simulink model "cartpole"  (R2019b)
settings: Solver=ode15s  StartTime=0.0  StopTime=10  MaxStep=0.01  RelTol=1e-3  EnableMultiTasking=on
values from neighbouring files (symbols this model uses):
  cartpole_init_pose = [-(ground.w/2-1) tire.r+ground.l/2 0]    [cartpole_conf.m]
  g = 9.81    [cartpole_conf.m]
  m_cart = body.m + 2*tire.m + 4*omni.m    [cartpole_conf.m]
  max_steer = 0.42    [cartpole_conf.m]
  max_v = 1    [cartpole_conf.m]
  path = [4.0 0.0 2.0]    [cartpole_conf.m]
  tread = tire.l + body.h    [cartpole_conf.m]
  waypoint_length = 0.05    [cartpole_conf.m]
undefined symbols (not defined in the file or in its folder): body, Body, ground, Ground, LBomni, LCtire, LFomni, omni, RBomni, RCtire, RFomni, sigbuilder_block, stick, Stick, tire, Wall1, Wall2, Wall3, Wall4, X, Y, Z
libraries: sm_lib x106, nesl_utility x18, simulink x5
(part 4 of 4)

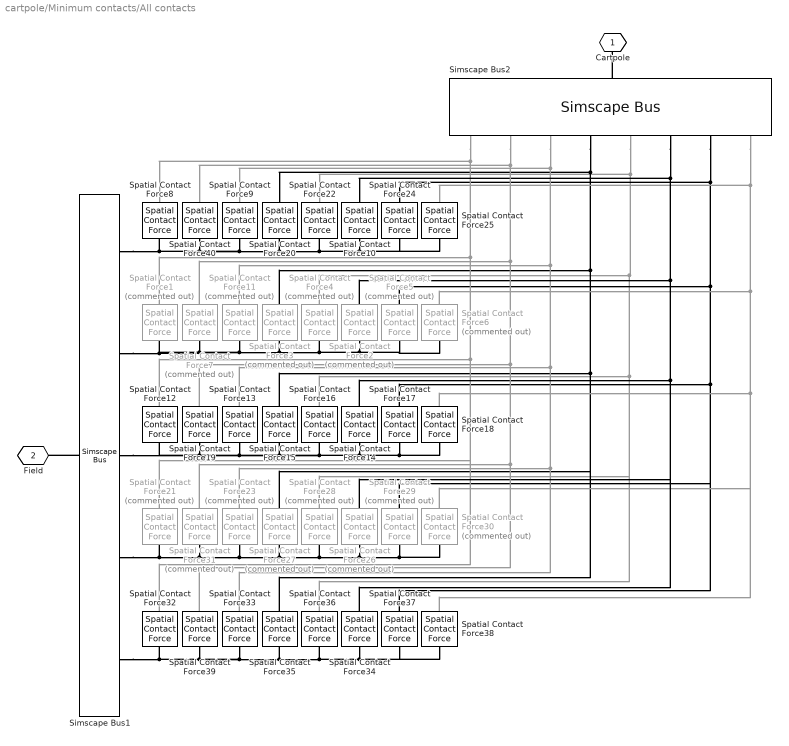
== system cartpole/Minimum contacts/All contacts ==
  Simscape Bus1 : SimscapeBus  HierarchyStrings=Wall1;Wall2;Wall3;Wall4;Ground
  Simscape Bus2 : SimscapeBus  HierarchyStrings=Stick;LFomni;LCtire;LBomni;RFomni;RCtire;RBomni;Body
  Spatial Contact Force{1..7,11,21,23,26..31} (16 alike) : sm_lib/Forces and Torques/Spatial Contact Force  Commented=on  CoefficientOfDynamicFriction=0.5  CoefficientOfStaticFriction=0.7  NormalDamping=1e3  NormalDampingUnits=N/(m/s)  NormalStiffness=1e6  NormalStiffnessUnits=N/m  FrictionalCriticalVelocity=1e-3  FrictionalCriticalVelocityUnits=m/s  SenseFrictionalForceMagnitude=off  SenseNormalForceMagnitude=off  SenseSeparationDistance=off  NormalTransitionRegionWidth=1e-4  NormalTransitionRegionWidthUnits=m  FrictionType=SmoothStickSlip
      settings: SourceProductName=Simscape Multibody
  Spatial Contact Force{8..10,12..20,22,24..25,32..40} (24 alike) : sm_lib/Forces and Torques/Spatial Contact Force  CoefficientOfDynamicFriction=0.5  CoefficientOfStaticFriction=0.7  NormalDamping=1e3  NormalDampingUnits=N/(m/s)  NormalStiffness=1e6  NormalStiffnessUnits=N/m  FrictionalCriticalVelocity=1e-3  FrictionalCriticalVelocityUnits=m/s  SenseFrictionalForceMagnitude=off  SenseNormalForceMagnitude=off  SenseSeparationDistance=off  NormalTransitionRegionWidth=1e-4  NormalTransitionRegionWidthUnits=m  FrictionType=SmoothStickSlip
      settings: SourceProductName=Simscape Multibody
  Cartpole : PMIOPort  Side=Right
  Field : PMIOPort  Port=2  Side=Left
  connections:
  Spatial Contact Force4/RConn1 -- Spatial Contact Force36/RConn1 -- Spatial Contact Force28/RConn1 -- Spatial Contact Force16/RConn1 -- Simscape Bus2/LConn5 -- Spatial Contact Force22/RConn1
  Spatial Contact Force1/LConn1 -- Simscape Bus1/LConn2 -- Spatial Contact Force7/LConn1 -- Spatial Contact Force11/LConn1 -- Spatial Contact Force3/LConn1 -- Spatial Contact Force2/LConn1 -- Spatial Contact Force6/LConn1 -- Spatial Contact Force5/LConn1 -- Spatial Contact Force4/LConn1
  Spatial Contact Force17/RConn1 -- Spatial Contact Force5/RConn1 -- Simscape Bus2/LConn7 -- Spatial Contact Force24/RConn1 -- Spatial Contact Force37/RConn1 -- Spatial Contact Force29/RConn1
  Spatial Contact Force15/RConn1 -- Spatial Contact Force3/RConn1 -- Simscape Bus2/LConn4 -- Spatial Contact Force20/RConn1 -- Spatial Contact Force35/RConn1 -- Spatial Contact Force27/RConn1
  Spatial Contact Force32/LConn1 -- Simscape Bus1/LConn5 -- Spatial Contact Force34/LConn1 -- Spatial Contact Force38/LConn1 -- Spatial Contact Force37/LConn1 -- Spatial Contact Force36/LConn1 -- Spatial Contact Force35/LConn1 -- Spatial Contact Force33/LConn1 -- Spatial Contact Force39/LConn1
  Spatial Contact Force6/RConn1 -- Spatial Contact Force38/RConn1 -- Spatial Contact Force30/RConn1 -- Spatial Contact Force18/RConn1 -- Simscape Bus2/LConn8 -- Spatial Contact Force25/RConn1
  Spatial Contact Force1/RConn1 -- Spatial Contact Force32/RConn1 -- Spatial Contact Force21/RConn1 -- Spatial Contact Force12/RConn1 -- Simscape Bus2/LConn1 -- Spatial Contact Force8/RConn1
  Spatial Contact Force23/RConn1 -- Spatial Contact Force11/RConn1 -- Simscape Bus2/LConn3 -- Spatial Contact Force9/RConn1 -- Spatial Contact Force13/RConn1 -- Spatial Contact Force33/RConn1
  Spatial Contact Force17/LConn1 -- Spatial Contact Force14/LConn1 -- Spatial Contact Force15/LConn1 -- Simscape Bus1/LConn3 -- Spatial Contact Force12/LConn1 -- Spatial Contact Force19/LConn1 -- Spatial Contact Force13/LConn1 -- Spatial Contact Force16/LConn1 -- Spatial Contact Force18/LConn1
  Spatial Contact Force14/RConn1 -- Spatial Contact Force2/RConn1 -- Simscape Bus2/LConn6 -- Spatial Contact Force10/RConn1 -- Spatial Contact Force34/RConn1 -- Spatial Contact Force26/RConn1
  Spatial Contact Force21/LConn1 -- Simscape Bus1/LConn4 -- Spatial Contact Force26/LConn1 -- Spatial Contact Force30/LConn1 -- Spatial Contact Force29/LConn1 -- Spatial Contact Force28/LConn1 -- Spatial Contact Force27/LConn1 -- Spatial Contact Force23/LConn1 -- Spatial Contact Force31/LConn1
  Spatial Contact Force31/RConn1 -- Spatial Contact Force7/RConn1 -- Simscape Bus2/LConn2 -- Spatial Contact Force40/RConn1 -- Spatial Contact Force19/RConn1 -- Spatial Contact Force39/RConn1
  Spatial Contact Force8/LConn1 -- Simscape Bus1/LConn1 -- Spatial Contact Force10/LConn1 -- Spatial Contact Force25/LConn1 -- Spatial Contact Force24/LConn1 -- Spatial Contact Force22/LConn1 -- Spatial Contact Force20/LConn1 -- Spatial Contact Force9/LConn1 -- Spatial Contact Force40/LConn1
  Simscape Bus2/RConn1 -- Cartpole/RConn1
  Simscape Bus1/RConn1 -- Field/RConn1

== matlab function cartpole/Controllers/Tire controller/calc_tire_velocity ==
  data: v_l output; v input; omega input; angle_diff input; v_r output; tread input
function [v_l, v_r] = calc_tire_v(v, omega, angle_diff, tread)
if angle_diff < 0
    v_r = v - tread*omega/2;
    v_l = v + tread*omega/2;
else
    v_r = v;
    v_l = v;
end

== matlab function cartpole/Controllers/calc_omega ==
  data: local_v input; sensor_angle input; sensor_x input; omega output; angle_diff output; sensor_z input; x_ref input; z_ref input; init_pose input; local_angle output; max_steer input
function [omega, angle_diff, local_angle] = calc_omega(local_v, sensor_angle, sensor_x, sensor_z, x_ref, z_ref, init_pose, max_steer)
x_local = x_ref - (sensor_x + init_pose(1));
z_local = z_ref - (sensor_z + init_pose(3));
local_angle = atan2(z_local, x_local) - sensor_angle;
%dist = sqrt( x_local^2 + z_local^2 );
omega = 2*local_v*sin(local_angle) / sqrt( x_local^2 + z_local^2 );
angle_diff = max_steer - abs(local_angle);

== matlab function cartpole/Controllers/Steer controller/MATLAB Function2 ==
  data: angle_diff input; delta output; local_angle input
function delta = calc_delta(angle_diff, local_angle)
if angle_diff > 0
    delta = -local_angle;
else
    delta = 0.0;
end

== matlab function cartpole/Controllers/Pole controller/MATLAB Function1 ==
  data: local_ax output; ax input; az input; angle input; local_az output
function [local_ax, local_az]= calc_local_a(ax, az, angle)
c = cos(angle);
s = sin(angle);
local_ax = ax*c + az*s;
local_az = -ax*s + az*c;

== matlab function cartpole/Controllers/MATLAB Function1 ==
  data: sensor_angle input; local_vx output; vx input; vz input
function local_vx = calc_local_v(sensor_angle, vx, vz)
local_vx = vx*cos(sensor_angle) + vz*sin(sensor_angle);

== matlab function cartpole/Controllers/Pole controller/MATLAB Function ==
  data: a_x input; a_z input; theta_x output; g input; h input; Mc input; Mo input; m input; L input; theta_z output
function [theta_x, theta_z]= calc_theta(a_x, a_z, g, h, Mc, Mo, m, L)
theta_z = a_x/g - a_x*h*(Mc + 4*Mo)/(m*L*sqrt(g*g+a_x*a_x));
theta_x = a_z/g - a_z*h*(Mc + 4*Mo)/(m*L*sqrt(g*g+a_z*a_z));

== matlab function cartpole/Sensor/calc_true_angle ==
  data: abs_angle input; angle output; vz input
function angle = calc_t_angle(abs_angle, vz)
if vz > 0
    angle = abs_angle;
else
    angle = -abs_angle;
end
